simulink model "State_space_simulation_and_modelling"  (R2023b)
settings: Solver=VariableStepAuto  StartTime=0.0  StopTime=100  RelTol=1e-3
values from neighbouring files (symbols this model uses):
  A = [3 -5 2 ... (first row only)    [Solution_tf_from_state_space.m]    (also in State_space_code.m = [0 1;-ks/m -kd/m])
  B = [5 ... (first row only)    [Solution_tf_from_state_space.m]    (also in State_space_code.m = [0; 1/m])
  C = [1 -4 3]    [Solution_tf_from_state_space.m]    (also in State_space_code.m = [1 0])
  Ci = eye(2,2)    [State_space_code.m]
  D = 0    [Solution_tf_from_state_space.m]    (also in State_space_code.m = [0])
  Di = [0;0]    [State_space_code.m]
  x0 = [0;0]    [State_space_code.m]
settings Model: Creator=HP  LastModifiedBy=HP

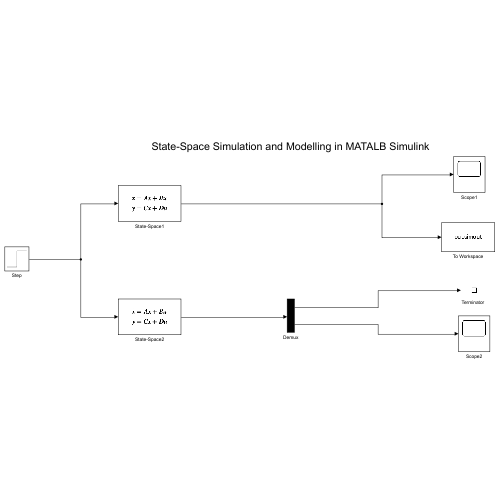
[thumbnail: Simulink's stored preview of the top-level diagram]
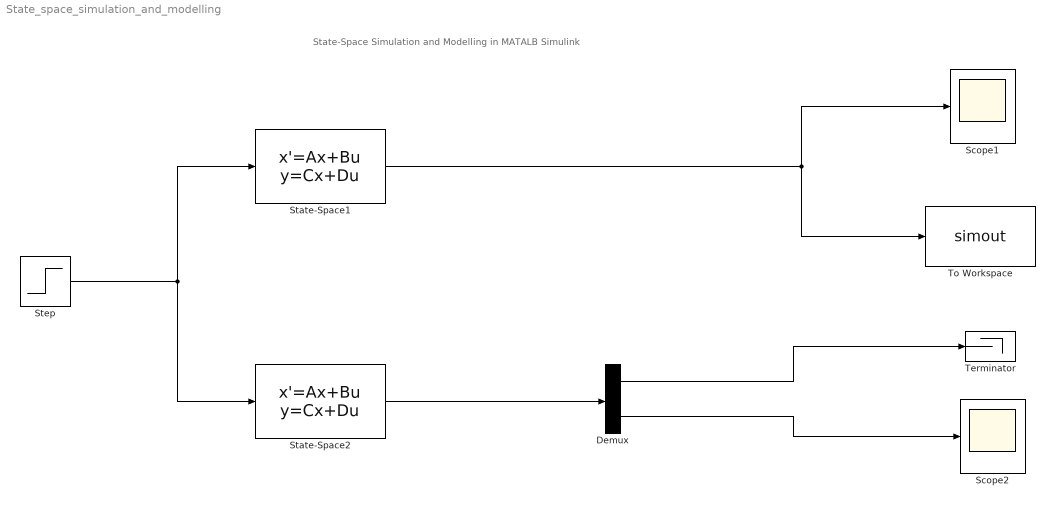
== system State_space_simulation_and_modelling ==
  note: State-Space Simulation and Modelling in MATALB Simulink
  Demux : Demux  Outputs=2
  Scope1 : Scope
  Scope2 : Scope
  State-Space1 : StateSpace  A=A  B=B  C=C  D=D  InitialCondition=x0
  State-Space2 : StateSpace  A=A  B=B  C=Ci  D=Di  InitialCondition=x0
  Step : Step  Time=0  SampleTime=0
  Terminator : Terminator
  To Workspace : ToWorkspace  VariableName=simout  SaveFormat=Timeseries  SampleTime=-1
  wires:
  Step/1 -> State-Space1/1, State-Space2/1
  State-Space1/1 -> Scope1/1, To Workspace/1
  State-Space2/1 -> Demux/1
  Demux/2 -> Scope2/1
  Demux/1 -> Terminator/1
